simulink model "sampleModel1801"  (R2023a)
settings: Solver=VariableStepAuto  StartTime=0.0  StopTime=10.0  RelTol=1e-3
libraries: hdlsllib x4, simulink x2
settings Model: Creator=user1  LastModifiedBy=user1

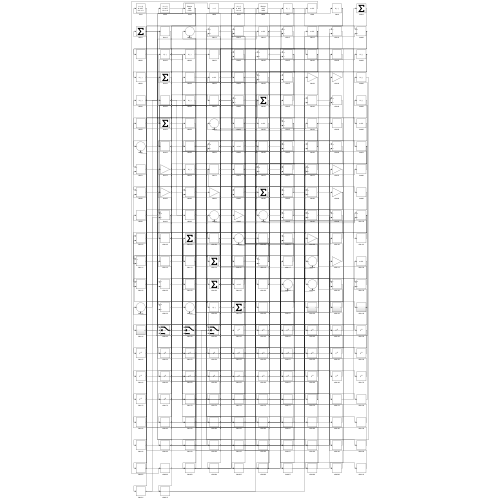
[thumbnail: Simulink's stored preview of the top-level diagram]
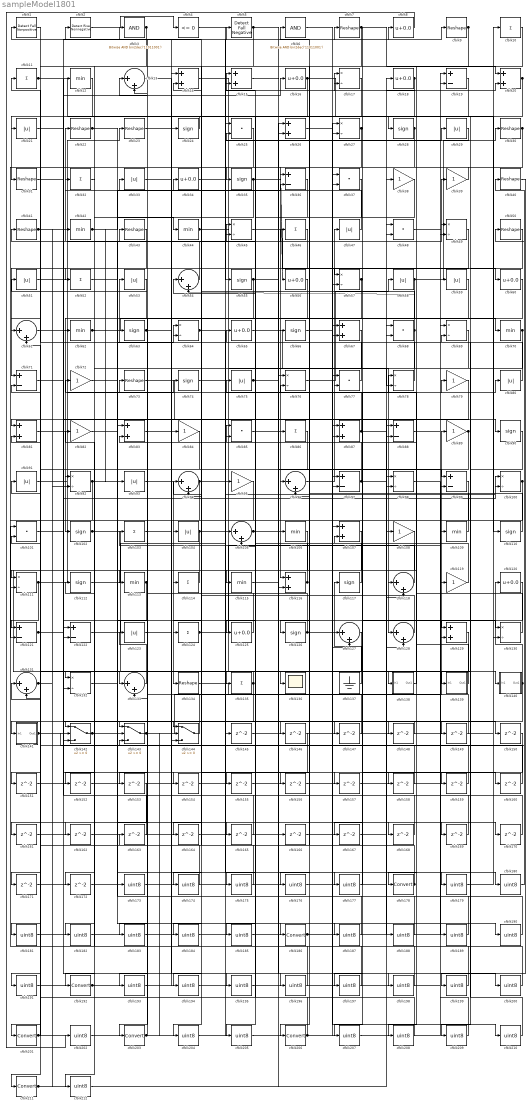
== system sampleModel1801 ==
  cfblk1 : hdlsllib/Logic and Bit Operations/Detect Fall Nonpositive  vinit=0  OutDataTypeStr=boolean
  cfblk{10..11,32,46,52,86,103,114,124,135} (10 alike) : Sum  Inputs=+
  cfblk{17,27,45,49,57,64,69,76,78,92,98,100,111,130,132} (15 alike) : Product  Inputs=*/  RndMeth=Zero  SaturateOnIntegerOverflow=on
  cfblk{25,37,48,68,77,85,101} (7 alike) : DotProduct  OutDataTypeStr=Inherit: Inherit via internal rule
  cfblk{24,28,35,55,63,66,74,90,102,110,112,117,126} (13 alike) : Signum
  cfblk{21,29,33,47,51,53,58..59,75,80,91,93,104,123} (14 alike) : Abs  SaturateOnIntegerOverflow=off
  cfblk{13,54,61,94,96,105,118,127..128,131,133} (11 alike) : Sum  Inputs=|++
  cfblk{12,42,44,62,70,106,109,113,115} (9 alike) : MinMax
  cfblk{14..15,20,26,67,81,83,87,107,116,129} (11 alike) : Sum
  cfblk{38..39,72,79,82,84,89,95,108,119} (10 alike) : Gain
  cfblk{8,16,18,34,56,60,65,120,125} (9 alike) : Bias  Bias=0.0  SaturateOnIntegerOverflow=off
  cfblk{19,36,71,88,97,99,121..122} (8 alike) : Sum  Inputs=+-
  cfblk{7,9,22..23,30..31,40..41,43,50,73,134} (12 alike) : Reshape
  cfblk136 : Scope
  cfblk137 : Ground
  cfblk138 : Subsystem
      settings: LibrarySourceBlock=|
      | hdlsllib/Ports &
      | Subsystems/Subsystem
  cfblk139 : Subsystem
      settings: LibrarySourceBlock=|
      | hdlsllib/Ports &
      | Subsystems/Subsystem
  cfblk140 : Subsystem
      settings: LibrarySourceBlock=|
      | hdlsllib/Ports &
      | Subsystems/Subsystem
  cfblk141 : Subsystem
      settings: LibrarySourceBlock=|
      | hdlsllib/Ports &
      | Subsystems/Subsystem
  cfblk142 : Switch  SaturateOnIntegerOverflow=off  InputSameDT=off
  cfblk143 : Switch  SaturateOnIntegerOverflow=off  InputSameDT=off
  cfblk144 : Switch  SaturateOnIntegerOverflow=off  InputSameDT=off
  cfblk{145..172} (28 alike) : Delay  SampleTime=1
  cfblk{173..177,179..185,187..191,193..200,202,204..205,207..210,212} (33 alike) : DataTypeConversion  OutDataTypeStr=uint8  SaturateOnIntegerOverflow=off  RndMeth=Floor
  cfblk{178,186,192,201,203,206,211} (7 alike) : DataTypeConversion  SaturateOnIntegerOverflow=off  RndMeth=Floor
  cfblk2 : hdlsllib/Logic and Bit Operations/Detect Rise Nonnegative  vinit=0  OutDataTypeStr=boolean
  cfblk3 : simulink/Logic and Bit Operations/Bitwise Operator  logicop=AND  UseBitMask=on  BitMask=bin2dec('11011001')  BitMaskRealWorld=Stored Integer
      settings: LibrarySourceBlock=|
      | hdlsllib/Logic and Bit
      | Operations/Bitwise
      | Operator
  cfblk4 : hdlsllib/Logic and Bit Operations/Compare To Zero  relop=<=  OutDataTypeStr=boolean
  cfblk5 : hdlsllib/Logic and Bit Operations/Detect Fall Negative  vinit=0  OutDataTypeStr=boolean
  cfblk6 : simulink/Logic and Bit Operations/Bitwise Operator  logicop=AND  UseBitMask=on  BitMask=bin2dec('11011001')  BitMaskRealWorld=Stored Integer
      settings: LibrarySourceBlock=|
      | hdlsllib/Logic and Bit
      | Operations/Bitwise
      | Operator
  wires:
  cfblk14/1 -> cfblk136/1
  cfblk134/1 -> cfblk89/1
  cfblk140/1(Out1) -> cfblk120/1, cfblk161/1
  cfblk110/1 -> cfblk34/1
  cfblk77/1 -> cfblk53/1
  cfblk111/1 -> cfblk23/1, cfblk121/1
  cfblk117/1 -> cfblk54/1
  cfblk10/1 -> cfblk178/1
  cfblk42/1 -> cfblk93/1, cfblk36/2
  cfblk122/1 -> cfblk130/1
  cfblk76/1 -> cfblk58/1
  cfblk116/1 -> cfblk75/1, cfblk41/1
  cfblk45/1 -> cfblk60/1
  cfblk62/1 -> cfblk70/1, cfblk92/1
  cfblk1/1 -> cfblk133/1
  cfblk36/1 -> cfblk116/1
  cfblk2/1 -> cfblk4/1
  cfblk43/1 -> cfblk71/1
  cfblk50/1 -> cfblk139/1(In1)
  cfblk44/1 -> cfblk128/1, cfblk17/1
  cfblk19/1 -> cfblk192/1
  cfblk9/1 -> cfblk66/1, cfblk151/1
  cfblk92/1 -> cfblk111/2, cfblk155/1
  cfblk127/1 -> cfblk203/1
  cfblk53/1 -> cfblk102/1
  cfblk135/1 -> cfblk132/1, cfblk171/1
  cfblk54/1 -> cfblk22/1
  cfblk139/1(Out1) -> cfblk85/1
  cfblk79/1 -> cfblk141/1(In1)
  cfblk103/1 -> cfblk24/1
  cfblk86/1 -> cfblk211/1
  cfblk138/1(Out1) -> cfblk78/1
  cfblk3/1 -> cfblk62/1, cfblk162/1
  cfblk11/1 -> cfblk28/1, cfblk154/1
  cfblk12/1 -> cfblk31/1
  cfblk24/1 -> cfblk21/1
  cfblk124/1 -> cfblk109/1, cfblk100/1, cfblk177/1
  cfblk137/1 -> cfblk117/1
  cfblk96/1 -> cfblk47/1
  cfblk102/1 -> cfblk138/1(In1), cfblk179/1
  cfblk38/1 -> cfblk206/1
  cfblk46/1 -> cfblk131/2
  cfblk74/1 -> cfblk29/1
  cfblk28/1 -> cfblk96/1, cfblk121/2
  cfblk47/1 -> cfblk33/1
  cfblk93/1 -> cfblk134/1
  cfblk131/1 -> cfblk91/1, cfblk92/2
  cfblk91/1 -> cfblk14/1
  cfblk104/1 -> cfblk80/1, cfblk142/3
  cfblk132/1 -> cfblk64/1
  cfblk142/1 -> cfblk45/1, cfblk146/1
  cfblk58/1 -> cfblk30/1, cfblk144/3
  cfblk75/1 -> cfblk115/1, cfblk149/1
  cfblk51/1 -> cfblk39/1
  cfblk21/1 -> cfblk143/1
  cfblk97/1 -> cfblk63/1, cfblk20/2
  cfblk70/1 -> cfblk126/1, cfblk164/1
  cfblk17/1 -> cfblk104/1
  cfblk20/1 -> cfblk124/1, cfblk159/1
  cfblk4/1 -> cfblk55/1
  cfblk130/1 -> cfblk72/1
  cfblk60/1 -> cfblk118/1
  cfblk55/1 -> cfblk168/1, cfblk193/1
  cfblk95/1 -> cfblk201/1
  cfblk84/1 -> cfblk143/2
  cfblk39/1 -> cfblk35/1
  cfblk6/1 -> cfblk97/1
  cfblk83/1 -> cfblk186/1
  cfblk5/1 -> cfblk61/1, cfblk99/1
  cfblk128/1 -> cfblk14/2
  cfblk109/1 -> cfblk65/1
  cfblk143/1 -> cfblk27/2, cfblk165/1
  cfblk27/1 -> cfblk36/1, cfblk147/1
  cfblk49/1 -> cfblk81/1
  cfblk41/1 -> cfblk12/1, cfblk3/1
  cfblk23/1 -> cfblk88/2
  cfblk65/1 -> cfblk78/2
  cfblk63/1 -> cfblk5/1, cfblk158/1
  cfblk106/1 -> cfblk135/1
  cfblk34/1 -> cfblk8/1
  cfblk7/1 -> cfblk20/1, cfblk57/1, cfblk174/1
  cfblk29/1 -> cfblk25/2
  cfblk18/1 -> cfblk57/2, cfblk17/2, cfblk185/1
  cfblk118/1 -> cfblk103/1
  cfblk119/1 -> cfblk32/1
  cfblk80/1 -> cfblk15/1
  cfblk89/1 -> cfblk167/1, cfblk194/1
  cfblk73/1 -> cfblk87/2
  cfblk30/1 -> cfblk144/1, cfblk96/2
  cfblk125/1 -> cfblk94/1
  cfblk48/1 -> cfblk49/1
  cfblk35/1 -> cfblk56/1, cfblk52/1
  cfblk68/1 -> cfblk54/2, cfblk2/1, cfblk182/1
  cfblk56/1 -> cfblk125/1
  cfblk94/1 -> cfblk142/2, cfblk79/1
  cfblk100/1 -> cfblk152/1, cfblk153/1
  cfblk113/1 -> cfblk132/2, cfblk172/1
  cfblk16/1 -> cfblk110/1, cfblk114/1
  cfblk114/1 -> cfblk111/1
  cfblk87/1 -> cfblk76/2, cfblk170/1
  cfblk112/1 -> cfblk7/1
  cfblk22/1 -> cfblk129/1, cfblk44/1
  cfblk144/1 -> cfblk51/1
  cfblk88/1 -> cfblk59/1
  cfblk71/1 -> cfblk90/1
  cfblk25/1 -> cfblk122/2
  cfblk105/1 -> cfblk200/1, cfblk205/1
  cfblk141/1(Out1) -> cfblk40/1, cfblk16/1
  cfblk81/1 -> cfblk74/1
  cfblk121/1 -> cfblk9/1, cfblk100/2
  cfblk126/1 -> cfblk43/1, cfblk210/1
  cfblk108/1 -> cfblk113/1
  cfblk133/1 -> cfblk123/1
  cfblk64/1 -> cfblk140/1(In1), cfblk129/2
  cfblk37/1 -> cfblk105/2
  cfblk78/1 -> cfblk11/1
  cfblk57/1 -> cfblk97/2, cfblk176/1
  cfblk66/1 -> cfblk128/2
  cfblk61/1 -> cfblk46/1
  cfblk145/1 -> cfblk130/2
  cfblk147/1 -> cfblk87/1
  cfblk115/1 -> cfblk148/1
  cfblk148/1 -> cfblk142/1
  cfblk149/1 -> cfblk1/1
  cfblk33/1 -> cfblk150/1
  cfblk151/1 -> cfblk105/1
  cfblk152/1 -> cfblk76/1
  cfblk154/1 -> cfblk49/2
  cfblk155/1 -> cfblk27/1
  cfblk59/1 -> cfblk156/1
  cfblk156/1 -> cfblk88/1
  cfblk85/1 -> cfblk157/1
  cfblk158/1 -> cfblk77/2
  cfblk159/1 -> cfblk81/2
  cfblk15/1 -> cfblk160/1
  cfblk160/1 -> cfblk143/3
  cfblk161/1 -> cfblk118/2
  cfblk162/1 -> cfblk116/2
  cfblk163/1 -> cfblk122/1
  cfblk164/1 -> cfblk45/2
  cfblk165/1 -> cfblk94/2
  cfblk166/1 -> cfblk37/2
  cfblk167/1 -> cfblk48/2
  cfblk168/1 -> cfblk68/1
  cfblk52/1 -> cfblk169/1
  cfblk169/1 -> cfblk25/1
  cfblk170/1 -> cfblk133/2
  cfblk171/1 -> cfblk106/1
  cfblk172/1 -> cfblk108/1
  cfblk82/1 -> cfblk173/1
  cfblk173/1 -> cfblk18/1
  cfblk174/1 -> cfblk82/1
  cfblk107/1 -> cfblk175/1
  cfblk175/1 -> cfblk61/2
  cfblk176/1 -> cfblk107/1
  cfblk177/1 -> cfblk107/2
  cfblk178/1 -> cfblk64/2, cfblk6/1
  cfblk179/1 -> cfblk10/1
  cfblk26/1 -> cfblk180/1
  cfblk180/1 -> cfblk50/1
  cfblk129/1 -> cfblk181/1
  cfblk181/1 -> cfblk26/1
  cfblk182/1 -> cfblk26/2
  cfblk67/1 -> cfblk183/1
  cfblk183/1 -> cfblk85/2
  cfblk99/1 -> cfblk184/1
  cfblk184/1 -> cfblk67/1
  cfblk185/1 -> cfblk67/2
  cfblk186/1 -> cfblk99/2, cfblk48/1
  cfblk123/1 -> cfblk187/1
  cfblk187/1 -> cfblk83/1
  cfblk157/1 -> cfblk188/1
  cfblk188/1 -> cfblk83/2
  cfblk98/1 -> cfblk189/1
  cfblk189/1 -> cfblk37/1
  cfblk72/1 -> cfblk190/1
  cfblk190/1 -> cfblk98/1
  cfblk153/1 -> cfblk191/1
  cfblk191/1 -> cfblk98/2
  cfblk192/1 -> cfblk166/1, cfblk84/1
  cfblk193/1 -> cfblk19/1
  cfblk194/1 -> cfblk19/2
  cfblk101/1 -> cfblk195/1
  cfblk195/1 -> cfblk77/1
  cfblk31/1 -> cfblk196/1
  cfblk196/1 -> cfblk101/1
  cfblk150/1 -> cfblk197/1
  cfblk197/1 -> cfblk101/2
  cfblk13/1 -> cfblk198/1
  cfblk198/1 -> cfblk112/1
  cfblk40/1 -> cfblk199/1
  cfblk199/1 -> cfblk13/1
  cfblk200/1 -> cfblk13/2
  cfblk201/1 -> cfblk119/1, cfblk71/2
  cfblk8/1 -> cfblk202/1
  cfblk202/1 -> cfblk95/1
  cfblk203/1 -> cfblk145/1, cfblk144/2, cfblk73/1
  cfblk146/1 -> cfblk204/1
  cfblk204/1 -> cfblk127/1
  cfblk205/1 -> cfblk127/2
  cfblk206/1 -> cfblk15/2, cfblk131/1
  cfblk120/1 -> cfblk207/1
  cfblk207/1 -> cfblk38/1
  cfblk69/1 -> cfblk208/1
  cfblk208/1 -> cfblk163/1
  cfblk90/1 -> cfblk209/1
  cfblk209/1 -> cfblk69/1
  cfblk210/1 -> cfblk69/2
  cfblk211/1 -> cfblk68/2, cfblk42/1
  cfblk32/1 -> cfblk212/1
  cfblk212/1 -> cfblk86/1

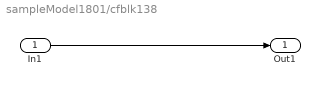
== system sampleModel1801/cfblk138 ==
  In1 : Inport
  Out1 : Outport
  wires:
  In1/1 -> Out1/1

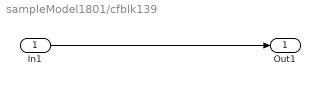
== system sampleModel1801/cfblk139 ==
  In1 : Inport
  Out1 : Outport
  wires:
  In1/1 -> Out1/1

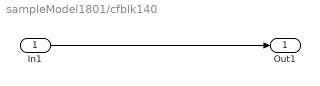
== system sampleModel1801/cfblk140 ==
  In1 : Inport
  Out1 : Outport
  wires:
  In1/1 -> Out1/1

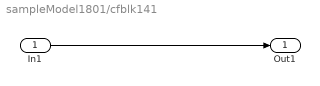
== system sampleModel1801/cfblk141 ==
  In1 : Inport
  Out1 : Outport
  wires:
  In1/1 -> Out1/1
